simulink model "sim_completa"  (Simulink 8.6)
settings: Solver=VariableStepAuto  StartTime=0.0  StopTime=25  FixedStep=0.01  RelTol=1e-3
undefined symbols (not defined in the file or in its folder): jib, jib_x0, jib_xref, tower, tower_x0, tower_xref, Ts
libraries: simulink x2, mpclib x2
settings Model: Creator=pdoren  LastModifiedBy=pdoren
settings DataIOCC: SaveFormat=Dataset  SignalLoggingSaveFormat=Dataset
settings OptimizationCC: ExpressionDepthLimit=128
settings DebuggingCC: UnderspecifiedInitializationDetection=Simplified  MergeDetectMultiDrivingBlocksExec=error  SolverPrmCheckMsg=none  FcnCallInpInsideContextMsg=EnableAllAsError  StateNameClashWarn=none
settings HardwareCC: ProdBitPerPointer=64  ProdLargestAtomicFloat=Float  ProdIntDivRoundTo=Zero  ProdEndianess=LittleEndian  ProdWordSize=64  ProdHWDeviceType=Intel->x86-64 (Windows64)
settings GRTTargetCC: GeneratePreprocessorConditionals=Use local settings  CombineOutputUpdateFcns=on  GRTInterface=off
settings ConfigComp: CovModelRefEnable=off

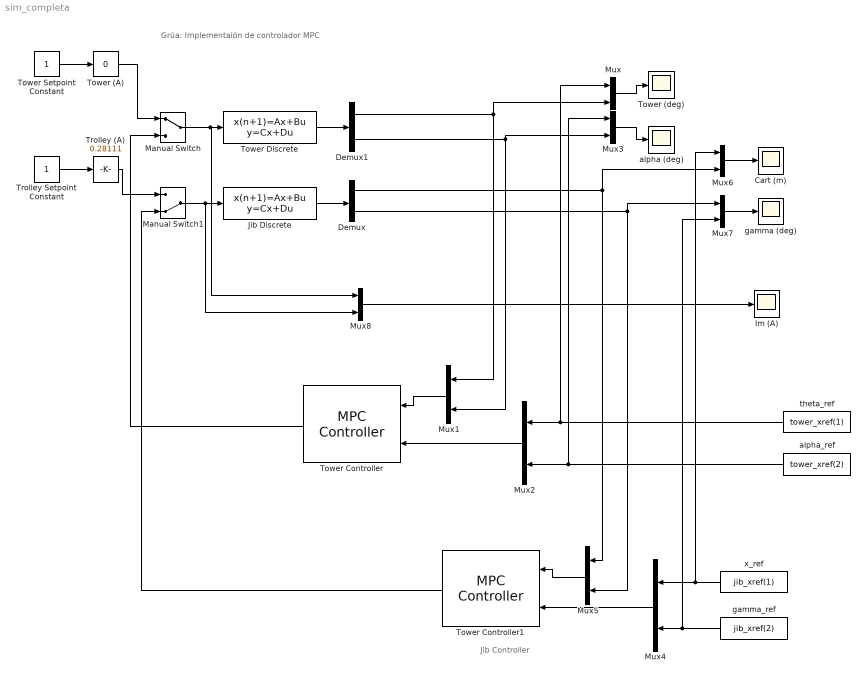
== system sim_completa ==
  note: Grúa: Implementaión de controlador MPC
  note: Jib Controller
  Cart (m) : Scope
  Demux : Demux  Outputs=2
  Demux1 : Demux  Outputs=2
  Im (A) : Scope
  Jib Discrete : DiscreteStateSpace  A=jib.A  B=jib.B  C=jib.C(jib.OutputGroup.MO,:)  D=jib.D(jib.OutputGroup.MO,:)  X0=jib_x0  SampleTime=Ts
  Manual Switch : ManualSwitch
  Manual Switch1 : ManualSwitch  CurrentSetting=0
  Mux{,1..8} (9 alike) : Mux  Inputs=2
  Tower (A) : simulink/Math Operations/Slider Gain  low=-0.5  gain=0  high=0.5
  Tower (deg) : Scope
  Tower Controller : mpclib/MPC Controller  mpcobj=tower_MPC  x0=[]  is_multiple=0  enable_value=0  return_u0=off  ref_from_ws=off  ref_signal_name=[]  ref_preview=on  md_from_ws=off  md_signal_name=[]  md_preview=on  from_project=off  project_file=MPCtask.mat  md_inport=off  mv_inport=off  cost_outport=off  return_sequence=off  return_qpstatus=off  return_state=off  state_inport=off  lims_inport=off  ywt_inport=off  is_designfromscratch=0  uwt_inport=off  duwt_inport=off  rhoeps_inport=off  uref_inport=off  n_ts=0.01  n_mv=1  n_md=0  n_ud=0  n_mo=2  n_uo=0  BlockDataType=double  SampleTimeInherited=off  switch_inport=off
  Tower Controller1 : mpclib/MPC Controller  mpcobj=jib_MPC  x0=[]  is_multiple=0  enable_value=0  return_u0=off  ref_from_ws=off  ref_signal_name=[]  ref_preview=on  md_from_ws=off  md_signal_name=[]  md_preview=on  from_project=off  project_file=MPCtask.mat  md_inport=off  mv_inport=off  cost_outport=off  return_sequence=off  return_qpstatus=off  return_state=off  state_inport=off  lims_inport=off  ywt_inport=off  is_designfromscratch=0  uwt_inport=off  duwt_inport=off  rhoeps_inport=off  uref_inport=off  n_ts=0.01  n_mv=1  n_md=0  n_ud=0  n_mo=2  n_uo=0  BlockDataType=double  SampleTimeInherited=off  switch_inport=off
  Tower Discrete : DiscreteStateSpace  A=tower.A  B=tower.B  C=tower.C(tower.OutputGroup.MO,:)  D=tower.D(tower.OutputGroup.MO,:)  X0=tower_x0  SampleTime=Ts
  "Tower Setpoint Constant " : Constant
  Trolley (A) : simulink/Math Operations/Slider Gain  low=-1  gain=0.28111  high=1
  "Trolley Setpoint Constant " : Constant
  alpha (deg) : Scope
  alpha_ref : Constant  Value=tower_xref(2)
  gamma (deg) : Scope
  gamma_ref : Constant  Value=jib_xref(2)
  theta_ref : Constant  Value=tower_xref(1)
  x_ref : Constant  Value=jib_xref(1)
  wires:
  Mux8/1 -> Im (A)/1
  Demux/2 -> Mux7/1, Mux5/2
  Demux/1 -> Mux6/2, Mux5/1
  Demux1/2 -> Mux3/2, Mux1/2
  Demux1/1 -> Mux/2, Mux1/1
  Mux1/1 -> Tower Controller/1
  theta_ref/1 -> Mux2/1, Mux/1
  Mux2/1 -> Tower Controller/2
  alpha_ref/1 -> Mux2/2, Mux3/1
  Mux/1 -> Tower (deg)/1
  Mux3/1 -> alpha (deg)/1
  "Tower Setpoint Constant "/1 -> Tower (A)/1
  Tower (A)/1 -> Manual Switch/1
  x_ref/1 -> Mux4/1, Mux6/1
  Mux4/1 -> Tower Controller1/2
  gamma_ref/1 -> Mux4/2, Mux7/2
  Mux5/1 -> Tower Controller1/1
  Mux6/1 -> Cart (m)/1
  Mux7/1 -> gamma (deg)/1
  "Trolley Setpoint Constant "/1 -> Trolley (A)/1
  Jib Discrete/1 -> Demux/1
  Tower Discrete/1 -> Demux1/1
  Manual Switch/1 -> Mux8/1, Tower Discrete/1
  Tower Controller/1 -> Manual Switch/2
  Trolley (A)/1 -> Manual Switch1/1
  Manual Switch1/1 -> Mux8/2, Jib Discrete/1
  Tower Controller1/1 -> Manual Switch1/2
